simulink model "transmission_fault_detection"  (R2022b)
settings: Solver=VariableStepAuto  StartTime=0.0  StopTime=Tend  RelTol=1e-3  AbsTol=1e-3
PreLoadFcn:
  | Tend= 40;
  | numClutches= 6;
  | g1= 1.6; % Planetary ring/sun gear ratio
  | g2= 2.35; % Ravigneaux ring/large sun gear ratio
  | g3= 2.65; % Ravigneaux ring/small sun gear ratio
  | 
  | clutch_DR_table= [...
  | 0	0	0	0	0	0	0
  | 0	0	0	0	0	1	0
  | 0	0	0	0	1	0	0
  | 0	0	0	0	1	1	0
  | 0	0	0	1	0	0	0
  | 0	0	0	1	0	1	0
  | 0	0	0	1	1	0	0
  | 0	0	0	1	1	1	0
  | 0	0	1	0	0	0	0.002917
  | 0	0	1	0	0	1	0.004564
  | 0	0	1	0	1	0	0.009493
  | 0	0	1	0	1	1	0.412308
  | 0	0	1	1	0	0	0.011091
  | 0	0	1	1	0	1	0.232221
  | 0	0	1	1	1	0	0
  | 0	1	0	0	0	0	0.012267
  | 0	1	0	0	0	1	0.009497
  | 0	1	0	0	1	0	1.425532
  | 0	1	0	0	1	1	1.425532
  | 0	1	1	0	0	0	0.095756
  | 0	1	1	0	0	1	0.854862
  | 0	1	1	0	1	0	1.425532
  | 1	0	0	0	0	0	0.0001000
  | 1	0	0	0	0	1	0.0001100
  | 1	0	0	0	1	0	0
  | 1	0	0	1	0	0	-0.009327
  | 1	0	0	1	0	1	-0.261866
  | 1	0	0	1	1	0	0
  | 1	0	1	0	0	0	0.005888
  | 1	0	1	0	0	1	0.615385
  | 1	0	1	0	1	0	0
  | 1	0	1	1	0	0	0
  | 1	1	0	0	0	0	0.116338
  | 1	1	0	0	0	1	1.163666
  | 1	1	0	0	1	0	1.425532
  | 1	1	1	0	0	0	1];
libraries: fl_lib x19, nesl_utility x10, sdl_lib x8, simulink x4, matrix_library x1
CloseFcn:
  | clear clutch_DR_table numClutches g1 g2 g3 Tend simlog_sdl_transmission_fault_detection
  | clear logsout yout tout
  | try,close(h1_sdl_transmission_fault_detection),end
  | clear h1_sdl_transmission_fault_detection
Description:
  | Transmission Fault Detection
settings Model: PauseTimes=1  Creator=The MathWorks, Inc.  LastModifiedBy=lwh
settings SolverCC: AutoScaleAbsTol=off  MaxConsecutiveZCs=100  AlgebraicLoopSolver=TrustRegion  MaxZcPerStep=1
settings DataIOCC: ReturnWorkspaceOutputs=off
settings DebuggingCC: UnconnectedInputMsg=warning  UnconnectedOutputMsg=warning  UnconnectedLineMsg=warning  SymbolicDimsDataTypeCodeGenerationDiagnostic=none  SFMachineParentedDataDiag=warning
settings ModelReferenceCC: EnableRefExpFcnMdlSchedulingChecks=on
settings SFSimCC: CustomCodeUndefinedFunction=UseInterfaceOnly
settings RTWCC: DLArmComputeVersion=19.05
settings SimscapeCC: SimscapeLogType=all  SimscapeLogSimulationStatistics=on  SimscapeLogName=simlog_transmission_fault_detection  SimscapeLogDataHistory=10000

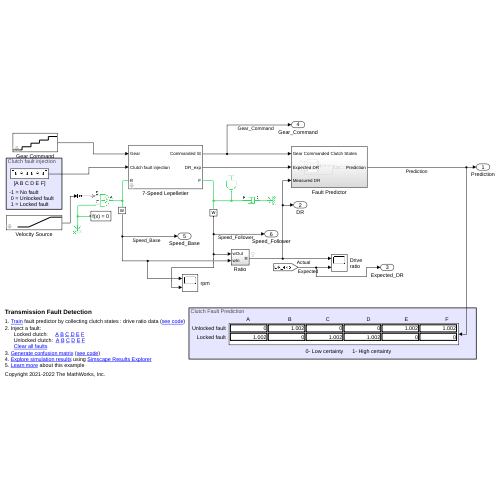
[thumbnail: Simulink's stored preview of the top-level diagram]
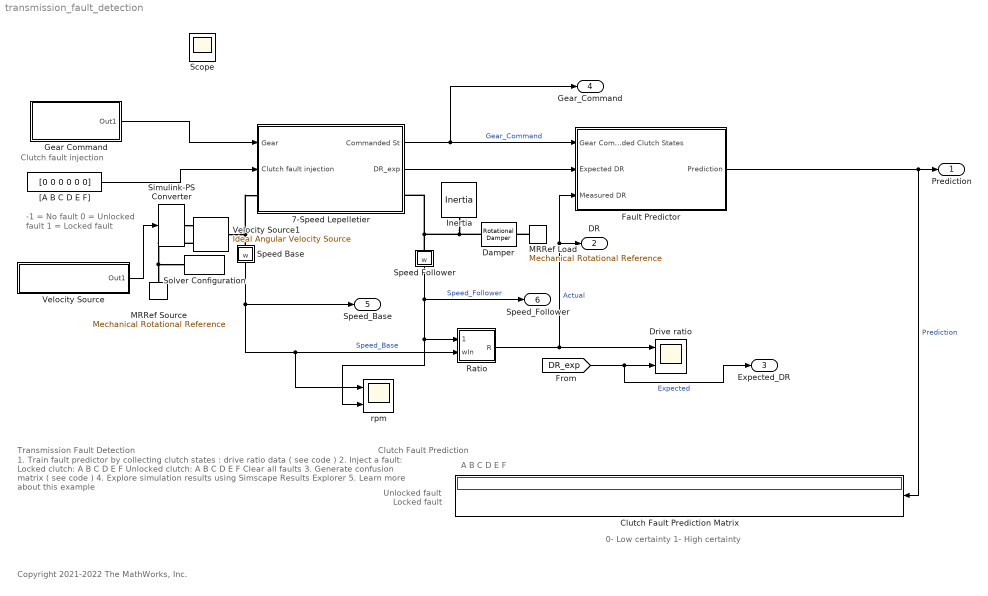
== system transmission_fault_detection ==
  note: Clutch fault injection
  note: -1 = No fault
      |  0 = Unlocked fault
      |  1 = Locked fault
  note: Locked fault
  note: 0- Low certainty 1- High certainty
  note: 1. Train fault predictor by collecting clutch states : drive ratio data ( see code )
      | 2. Inject a fault:
      | Locked clutch: A B C D E F
      | Unlocked clutch: A B C D E F
      | Clear all faults
      | 3. Generate confusion matrix ( see code )
      | 4. Explore simulation results using Simscape Results Explorer
      | 5. Learn more about this example
  note: A B C D E F
  note: Unlocked fault
  note: Transmission Fault Detection
  note: Clutch Fault Prediction
  note: Copyright 2021-2022 The MathWorks, Inc.
  7-Speed Lepelletier : Subsystem  mask(7-Speed Lepelletier){InitGear=Neutral, ShowInLibBrowser=0, ClutchSchedule={[0 1 0 0 1 1];[1 1 0 0 0 1];[1 1 1 0 0 0];[0 1 1 0 0 1];[1 0 1 0 0 1];[0 0 1 0 1 1];[0 0 1 1 0 1];[1 0 0 1 0 1];[0 0 0 1 0 1]}}
      mask prompts: InitGear "Initial gear"
      mask help: physmod:sdl:library:transmissions:SevenSpeedLepelletier
      mask init:
      | set_param([gcb,'/Clutch A'],'initial_state_locked',num2str(ClutchSchedule{InitGear}(1)));
      | set_param([gcb,'/Clutch B'],'initial_state_locked',num2str(ClutchSchedule{InitGear}(2)));
      | set_param([gcb,'/Clutch C'],'initial_state_locked',num2str(ClutchSchedule{InitGear}(3)));
      | set_param([gcb,'/Clutch D'],'initial_state_locked',num2str(ClutchSchedule{InitGear}(4)));
      | set_param([gcb,'/Clutch E'],'initial_state_locked',num2str(ClutchSchedule{InitGear}(5)));
      | set_param([gcb,'/Clutch F'],'initial_state_locked',num2str(ClutchSchedule{InitGear}(6)));
      mask Help: web([docroot '/sdl/ref/7speedlepelletier.html'])
      mask TypeOptions InitGear: 7 | 6 | 5 | 4 | 3 | 2 | 1 | physmod:sdl:library:transmissions:Reverse | physmod:sdl:library:transmissions:Neutral
  Clutch Fault Prediction Matrix : Display
  Damper : fl_lib/Mechanical/Rotational Elements/Rotational Damper  D=5 N*m/(rad/s)  w_specify=off  w_priority=High  w=0 rad/s  w_nominal_specify=off  w_nominal_unit=rad/s  w_nominal_value=1  t_specify=off  t_priority=High  t=0 N*m  t_nominal_specify=off  t_nominal_unit=N*m  t_nominal_value=1
  Drive ratio : Scope  NumInputPorts=2
  Fault Predictor : Subsystem
  Gear Command : Subsystem  mask{Repeating_Sequence=[7 7 7 7 7 7 7 7 7 7 7], Sample_time=4}
      mask prompts: Repeating_Sequence "Output"; Sample_time "Sample time"
      mask Display:
      | plot(0, -10)
      | plot(100, 100)
      | plot([0 20 20 40 40 60 60 80 80 100], [0 0 20 20 40 40 60 60 80 80]);
  Inertia : fl_lib/Mechanical/Rotational Elements/Inertia  inertia=.01 kg*m^2  num_ports=foundation.enum.numPorts2.one  w_specify=off  w_priority=High  w=0 rad/s  w_nominal_specify=off  w_nominal_unit=rad/s  w_nominal_value=1  t_specify=off  t_priority=High  t=0 N*m  t_nominal_specify=off  t_nominal_unit=N*m  t_nominal_value=1
  MRRef Load : fl_lib/Mechanical/Rotational Elements/Mechanical Rotational Reference
  MRRef Source : fl_lib/Mechanical/Rotational Elements/Mechanical Rotational Reference
  Ratio : Subsystem
  Simulink-PS Converter : nesl_utility/Simulink-PS Converter  PhysicalDomain=network_engine_domain  SubClassName=ps_input  LeftPortType=input  RightPortType=output  PseudoPeriodic=off  Frequencies=[]  NoiseDistribution=none  NoiseParameters=[]  Unit=rpm  AffineConversion=off  FilteringAndDerivatives=filter  SimscapeFilterOrder=1  InputFilterTimeConstant=0.001  UdotUserProvided=1
  Solver Configuration : nesl_utility/Solver Configuration  PhysicalDomain=network_engine_domain  SubClassName=solver  LeftPortType=input  RightPortType=generic  Tones=[]  Harmonics=[]  SimulateNoise=off  Profile=off  UseLocalSampling=off  EnableSwitchedLinearOptims=on  FrequencyDomain=off  UseCCode=off  RelTol=0.001  AbsTol=1e-06  MinStep=1e-09  ToWorkspace=off  RevertToSquareIcSolve=off  NumHomotopyIterations=100  PhasorMode=off  PhasorModeNumHarmonics=1  ConsistencySolver=NEWTON_XTOL_AFTER_FTOL  IndexReductionMethod=DerivativeReplacement  DoDC=on  ResidualTolerance=1e-9  ConsistencyTolSource=GLOBAL  ConsistencyAbsTol=0.001  ConsistencyRelTol=0.001  ConsistencyTolFactor=0.001  UseLocalSolver=off  LocalSolverChoice=NE_PARTITIONING_ADVANCER  ResolveIndetEquations=on  FunctionEvalNumThread=1  LocalSolverSampleTime=0.001  DoFixedCost=off  MaxNonlinIter=3  MaxModeIter=2  ComputeImpulses=off  ImpulseIterations=2  LinearAlgebra=auto  LinearAlgebraNumThread=0  EquationFormulation=NE_TIME_EF  DelaysMemoryBudget=1024  AutomaticFiltering=on  FilteringTimeConstant=0.001  PartitionStorageMethod=EXHAUSTIVE  PartitionMemoryBudget=1024  PartitionMethod=ROBUST
  Speed Base : Subsystem
      mask Display: disp('w')
  Speed Follower : Subsystem
      mask Display: disp('w')
  Velocity Source1 : fl_lib/Mechanical/Mechanical Sources/Ideal Angular Velocity Source
  Velocity Source : Subsystem  VariantControl=Ramp  mask{slope=100, start=0.1, initial_speed=450, final_speed=450}
      mask prompts: slope "Slope (rpm/s)"; start "Start time (sec)"; initial_speed "Initial speed (rpm)"; final_speed "Final speed (rpm)"
      mask Display:
      | plot(0, 0)
      | plot(100, 100)
      | plot([20 40 80 100], [20 20 90 90]);
  "[A B C D E F]" : Constant  Value=[0 0 0 0 0 0]  VectorParams1D=off
  rpm : Scope  NumInputPorts=2
  Prediction : Outport
  DR : Outport  Port=2
  Expected_DR : Outport  Port=3
  Gear_Command : Outport  Port=4
  Speed_Base : Outport  Port=5
  Speed_Follower : Outport  Port=6
  Scope : Scope
  wires:
  Fault Predictor/1(Prediction) -> Prediction/1, Clutch Fault Prediction Matrix/1  "Prediction"
  7-Speed Lepelletier/2(DR_exp) -> Fault Predictor/2(Expected DR)
  7-Speed Lepelletier/1(Commanded St) -> Gear_Command/1, Fault Predictor/1(Gear Commanded Clutch States)  "Gear_Command"
  Speed Base/1(w) -> Speed_Base/1, rpm/1, Ratio/2(wIn)  "Speed_Base"
  Speed Follower/1(w) -> Speed_Follower/1, rpm/2, Ratio/1(wOut)  "Speed_Follower"
  "[A B C D E F]"/1 -> 7-Speed Lepelletier/2(Clutch fault injection)
  Ratio/1(R) -> DR/1, Fault Predictor/3(Measured DR), Drive ratio/1  "Actual"
  [DR_exp] -> Expected_DR/1, Drive ratio/2  "Expected"
  Velocity Source/1(Out1) -> Simulink-PS Converter/1
  Gear Command/1(Out1) -> 7-Speed Lepelletier/1(Gear)
  connections:
  Velocity Source1/RConn2 -- MRRef Source/LConn1 -- Solver Configuration/RConn1
  Damper/LConn1 -- Inertia/LConn1 -- Speed Follower/LConn1 -- 7-Speed Lepelletier/RConn1
  Speed Base/LConn1 -- 7-Speed Lepelletier/LConn1 -- Velocity Source1/LConn1
  Simulink-PS Converter/RConn1 -- Velocity Source1/RConn1
  MRRef Load/LConn1 -- Damper/RConn1

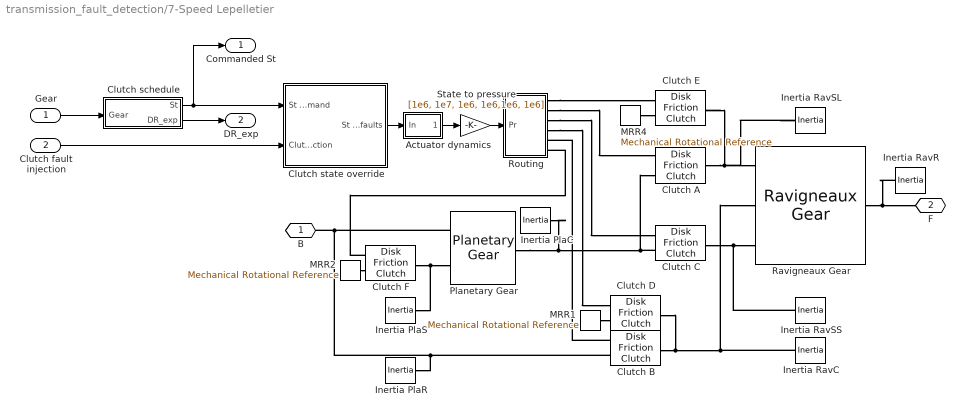
== system transmission_fault_detection/7-Speed Lepelletier ==
  Gear : Inport
  Clutch fault injection : Inport  Port=2
  Actuator dynamics : Subsystem  mask(First-order lag supporting vector signals){b=[1 1 1 1 1 1]*0.05, x_initial=ClutchSchedule{InitGear}}
      mask prompts: b "Filter time constant"; x_initial "Initial output"
      mask help: Models a lag of the form 1/(b*s+1) where s is the Laplace operator.
  Clutch schedule : Subsystem
  Clutch A : sdl_lib/Clutches/Disk Friction Clutch  geometry_model=2  r_eff=130 mm  d_o=150 mm  d_i=100 mm  nS=4  piston_area=0.001 m^2  unidirectional=0  friction_model=1  mu_w_vector=[ 0 0.1 0.2 0.3 0.4 0.5 1 2 5 10 100 1000 ] rad/s  temperature_TLU=[280.0, 300.0, 320.0] K  mu_static=0.65  mu_static_vector=[0.4, 0.38, 0.36]  mu_coulomb=0.6  mu_coulomb_vector=[ 0.29 0.28 0.26 0.22 0.21 0.2 0.2 0.19 0.19 0.19 0.19 0.19 ]  mu_coulomb_temp_vector=[0.3, 0.28, 0.25]  mu_coulomb_matrix=[0.34, 0.32, 0.3; 0.3, 0.28, 0.25; 0.25, 0.2, 0.15]  mu_interp_method=1  mu_extrap_method=1  d_f=1  w_tol=0.001 rad/s  pressure_min=100 Pa  mu_visc=0 N*m/(rad/s)  initial_state_locked=0  enable_faults=simscape.enum.onoff.off  fault_type=sdl.enum.clutchFault.lock  external_fault=simscape.enum.onoff.on  temporal_fault=simscape.enum.onoff.off  fault_time=5 s  report_fault=simscape.enum.assert.action.none  thermal_mass=25 kJ/K  T_init=300 K
      settings: InternalSimscapePortConfiguration="{\"Bottom\":[],\"Left\":[{\"id\":\"P\",\"label\":\"P\",\"type\":\"input\"},{\"id\":\"B\",\"label\":\"B\",\"type\":\"foundation.mechanical.rotational.rotational\"}],\"Right\":[{\"id\":\"F\",\"label\":\"F\",\"type\":\"foundation.mechanical.rotational.rotational\"}],\"Top\":[]}"
  Clutch B : sdl_lib/Clutches/Disk Friction Clutch  geometry_model=2  r_eff=130 mm  d_o=150 mm  d_i=100 mm  nS=4  piston_area=0.001 m^2  unidirectional=0  friction_model=1  mu_w_vector=[ 0 0.1 0.2 0.3 0.4 0.5 1 2 5 10 100 1000 ] rad/s  temperature_TLU=[280.0, 300.0, 320.0] K  mu_static=0.65  mu_static_vector=[0.4, 0.38, 0.36]  mu_coulomb=0.6  mu_coulomb_vector=[ 0.29 0.28 0.26 0.22 0.21 0.2 0.2 0.19 0.19 0.19 0.19 0.19 ]  mu_coulomb_temp_vector=[0.3, 0.28, 0.25]  mu_coulomb_matrix=[0.34, 0.32, 0.3; 0.3, 0.28, 0.25; 0.25, 0.2, 0.15]  mu_interp_method=1  mu_extrap_method=1  d_f=1  w_tol=0.001 rad/s  pressure_min=100 Pa  mu_visc=0 N*m/(rad/s)  initial_state_locked=0  enable_faults=simscape.enum.onoff.off  fault_type=sdl.enum.clutchFault.lock  external_fault=simscape.enum.onoff.off  temporal_fault=simscape.enum.onoff.off  fault_time=5 s  report_fault=simscape.enum.assert.action.none  thermal_mass=25 kJ/K  T_init=300 K
      settings: InternalSimscapePortConfiguration="{\"Bottom\":[],\"Left\":[{\"id\":\"P\",\"label\":\"P\",\"type\":\"input\"},{\"id\":\"B\",\"label\":\"B\",\"type\":\"foundation.mechanical.rotational.rotational\"}],\"Right\":[{\"id\":\"F\",\"label\":\"F\",\"type\":\"foundation.mechanical.rotational.rotational\"}],\"Top\":[]}"
  Clutch C : sdl_lib/Clutches/Disk Friction Clutch  geometry_model=2  r_eff=130 mm  d_o=150 mm  d_i=100 mm  nS=4  piston_area=0.001 m^2  unidirectional=0  friction_model=1  mu_w_vector=[ 0 0.1 0.2 0.3 0.4 0.5 1 2 5 10 100 1000 ] rad/s  temperature_TLU=[280.0, 300.0, 320.0] K  mu_static=0.65  mu_static_vector=[0.4, 0.38, 0.36]  mu_coulomb=0.6  mu_coulomb_vector=[ 0.29 0.28 0.26 0.22 0.21 0.2 0.2 0.19 0.19 0.19 0.19 0.19 ]  mu_coulomb_temp_vector=[0.3, 0.28, 0.25]  mu_coulomb_matrix=[0.34, 0.32, 0.3; 0.3, 0.28, 0.25; 0.25, 0.2, 0.15]  mu_interp_method=1  mu_extrap_method=1  d_f=1  w_tol=0.001 rad/s  pressure_min=100 Pa  mu_visc=0 N*m/(rad/s)  initial_state_locked=0  enable_faults=simscape.enum.onoff.off  fault_type=sdl.enum.clutchFault.lock  external_fault=simscape.enum.onoff.off  temporal_fault=simscape.enum.onoff.off  fault_time=5 s  report_fault=simscape.enum.assert.action.none  thermal_mass=25 kJ/K  T_init=300 K
      settings: InternalSimscapePortConfiguration="{\"Bottom\":[],\"Left\":[{\"id\":\"P\",\"label\":\"P\",\"type\":\"input\"},{\"id\":\"B\",\"label\":\"B\",\"type\":\"foundation.mechanical.rotational.rotational\"}],\"Right\":[{\"id\":\"F\",\"label\":\"F\",\"type\":\"foundation.mechanical.rotational.rotational\"}],\"Top\":[]}"
  Clutch D : sdl_lib/Clutches/Disk Friction Clutch  geometry_model=2  r_eff=130 mm  d_o=150 mm  d_i=100 mm  nS=4  piston_area=0.001 m^2  unidirectional=0  friction_model=1  mu_w_vector=[ 0 0.1 0.2 0.3 0.4 0.5 1 2 5 10 100 1000 ] rad/s  temperature_TLU=[280.0, 300.0, 320.0] K  mu_static=0.65  mu_static_vector=[0.4, 0.38, 0.36]  mu_coulomb=0.6  mu_coulomb_vector=[ 0.29 0.28 0.26 0.22 0.21 0.2 0.2 0.19 0.19 0.19 0.19 0.19 ]  mu_coulomb_temp_vector=[0.3, 0.28, 0.25]  mu_coulomb_matrix=[0.34, 0.32, 0.3; 0.3, 0.28, 0.25; 0.25, 0.2, 0.15]  mu_interp_method=1  mu_extrap_method=1  d_f=1  w_tol=0.001 rad/s  pressure_min=100 Pa  mu_visc=0 N*m/(rad/s)  initial_state_locked=1  enable_faults=simscape.enum.onoff.off  fault_type=sdl.enum.clutchFault.lock  external_fault=simscape.enum.onoff.off  temporal_fault=simscape.enum.onoff.off  fault_time=5 s  report_fault=simscape.enum.assert.action.none  thermal_mass=25 kJ/K  T_init=300 K
      settings: InternalSimscapePortConfiguration="{\"Bottom\":[],\"Left\":[{\"id\":\"P\",\"label\":\"P\",\"type\":\"input\"},{\"id\":\"B\",\"label\":\"B\",\"type\":\"foundation.mechanical.rotational.rotational\"}],\"Right\":[{\"id\":\"F\",\"label\":\"F\",\"type\":\"foundation.mechanical.rotational.rotational\"}],\"Top\":[]}"
  Clutch E : sdl_lib/Clutches/Disk Friction Clutch  geometry_model=2  r_eff=130 mm  d_o=150 mm  d_i=100 mm  nS=4  piston_area=0.001 m^2  unidirectional=0  friction_model=1  mu_w_vector=[ 0 0.1 0.2 0.3 0.4 0.5 1 2 5 10 100 1000 ] rad/s  temperature_TLU=[280.0, 300.0, 320.0] K  mu_static=0.65  mu_static_vector=[0.4, 0.38, 0.36]  mu_coulomb=0.6  mu_coulomb_vector=[ 0.29 0.28 0.26 0.22 0.21 0.2 0.2 0.19 0.19 0.19 0.19 0.19 ]  mu_coulomb_temp_vector=[0.3, 0.28, 0.25]  mu_coulomb_matrix=[0.34, 0.32, 0.3; 0.3, 0.28, 0.25; 0.25, 0.2, 0.15]  mu_interp_method=1  mu_extrap_method=1  d_f=1  w_tol=0.001 rad/s  pressure_min=100 Pa  mu_visc=0 N*m/(rad/s)  initial_state_locked=0  enable_faults=simscape.enum.onoff.off  fault_type=sdl.enum.clutchFault.lock  external_fault=simscape.enum.onoff.off  temporal_fault=simscape.enum.onoff.off  fault_time=5 s  report_fault=simscape.enum.assert.action.none  thermal_mass=25 kJ/K  T_init=300 K
      settings: InternalSimscapePortConfiguration="{\"Bottom\":[],\"Left\":[{\"id\":\"P\",\"label\":\"P\",\"type\":\"input\"},{\"id\":\"B\",\"label\":\"B\",\"type\":\"foundation.mechanical.rotational.rotational\"}],\"Right\":[{\"id\":\"F\",\"label\":\"F\",\"type\":\"foundation.mechanical.rotational.rotational\"}],\"Top\":[]}"
  Clutch F : sdl_lib/Clutches/Disk Friction Clutch  geometry_model=2  r_eff=130 mm  d_o=150 mm  d_i=100 mm  nS=4  piston_area=0.001 m^2  unidirectional=0  friction_model=1  mu_w_vector=[ 0 0.1 0.2 0.3 0.4 0.5 1 2 5 10 100 1000 ] rad/s  temperature_TLU=[280.0, 300.0, 320.0] K  mu_static=0.65  mu_static_vector=[0.4, 0.38, 0.36]  mu_coulomb=0.6  mu_coulomb_vector=[ 0.29 0.28 0.26 0.22 0.21 0.2 0.2 0.19 0.19 0.19 0.19 0.19 ]  mu_coulomb_temp_vector=[0.3, 0.28, 0.25]  mu_coulomb_matrix=[0.34, 0.32, 0.3; 0.3, 0.28, 0.25; 0.25, 0.2, 0.15]  mu_interp_method=1  mu_extrap_method=1  d_f=1  w_tol=0.001 rad/s  pressure_min=100 Pa  mu_visc=0 N*m/(rad/s)  initial_state_locked=1  enable_faults=simscape.enum.onoff.off  fault_type=sdl.enum.clutchFault.lock  external_fault=simscape.enum.onoff.off  temporal_fault=simscape.enum.onoff.off  fault_time=5 s  report_fault=simscape.enum.assert.action.none  thermal_mass=25 kJ/K  T_init=300 K
      settings: InternalSimscapePortConfiguration="{\"Bottom\":[],\"Left\":[{\"id\":\"P\",\"label\":\"P\",\"type\":\"input\"},{\"id\":\"B\",\"label\":\"B\",\"type\":\"foundation.mechanical.rotational.rotational\"}],\"Right\":[{\"id\":\"F\",\"label\":\"F\",\"type\":\"foundation.mechanical.rotational.rotational\"}],\"Top\":[]}"
  Clutch state override : Subsystem
  Inertia PlaC : fl_lib/Mechanical/Rotational Elements/Inertia  inertia=0.03 kg*m^2  num_ports=foundation.enum.numPorts2.one  w_specify=off  w_priority=High  w=0 rad/s  w_nominal_specify=off  w_nominal_unit=rad/s  w_nominal_value=1  t_specify=off  t_priority=High  t=0 N*m  t_nominal_specify=off  t_nominal_unit=N*m  t_nominal_value=1
  "Inertia PlaR " : fl_lib/Mechanical/Rotational Elements/Inertia  inertia=0.025 kg*m^2  num_ports=foundation.enum.numPorts2.one  w_specify=off  w_priority=High  w=0 rad/s  w_nominal_specify=off  w_nominal_unit=rad/s  w_nominal_value=1  t_specify=off  t_priority=High  t=0 N*m  t_nominal_specify=off  t_nominal_unit=N*m  t_nominal_value=1
  Inertia PlaS : fl_lib/Mechanical/Rotational Elements/Inertia  inertia=0.04 kg*m^2  num_ports=foundation.enum.numPorts2.one  w_specify=off  w_priority=High  w=0 rad/s  w_nominal_specify=off  w_nominal_unit=rad/s  w_nominal_value=1  t_specify=off  t_priority=High  t=0 N*m  t_nominal_specify=off  t_nominal_unit=N*m  t_nominal_value=1
  Inertia RavC : fl_lib/Mechanical/Rotational Elements/Inertia  inertia=0.03 kg*m^2  num_ports=foundation.enum.numPorts2.one  w_specify=off  w_priority=High  w=0 rad/s  w_nominal_specify=off  w_nominal_unit=rad/s  w_nominal_value=1  t_specify=off  t_priority=High  t=0 N*m  t_nominal_specify=off  t_nominal_unit=N*m  t_nominal_value=1
  Inertia RavR : fl_lib/Mechanical/Rotational Elements/Inertia  inertia=0.03 kg*m^2  num_ports=foundation.enum.numPorts2.one  w_specify=off  w_priority=High  w=0 rad/s  w_nominal_specify=off  w_nominal_unit=rad/s  w_nominal_value=1  t_specify=off  t_priority=High  t=0 N*m  t_nominal_specify=off  t_nominal_unit=N*m  t_nominal_value=1
  Inertia RavSL : fl_lib/Mechanical/Rotational Elements/Inertia  inertia=0.05 kg*m^2  num_ports=foundation.enum.numPorts2.one  w_specify=off  w_priority=High  w=0 rad/s  w_nominal_specify=off  w_nominal_unit=rad/s  w_nominal_value=1  t_specify=off  t_priority=High  t=0 N*m  t_nominal_specify=off  t_nominal_unit=N*m  t_nominal_value=1
  Inertia RavSS : fl_lib/Mechanical/Rotational Elements/Inertia  inertia=0.02 kg*m^2  num_ports=foundation.enum.numPorts2.one  w_specify=off  w_priority=High  w=0 rad/s  w_nominal_specify=off  w_nominal_unit=rad/s  w_nominal_value=1  t_specify=off  t_priority=High  t=0 N*m  t_nominal_specify=off  t_nominal_unit=N*m  t_nominal_value=1
  MRR1 : fl_lib/Mechanical/Rotational Elements/Mechanical Rotational Reference
  MRR2 : fl_lib/Mechanical/Rotational Elements/Mechanical Rotational Reference
  MRR4 : fl_lib/Mechanical/Rotational Elements/Mechanical Rotational Reference
  Planetary Gear : sdl_lib/Gears/Planetary Gear  rs_ratio=g1  friction_model=1  efficiency=[ 0.96 0.98 ]  temperature_TLU=[ 280 300 320 ] K  efficiency_sp_TLU=[ 0.95 0.9 0.85 ]  efficiency_rp_TLU=[ 0.95 0.9 0.85 ]  pwr_thr=[ 0.001 0.001 ] W  mu_visc=[ 0 0 ] N*m/(rad/s)  model_inertia=0  planet_inertia=0.001 kg*m^2  thermal_mass=50 J/K  T_init=300 K
  Ravigneaux Gear : sdl_lib/Gears/Ravigneaux Gear  rsl_ratio=g2  rss_ratio=g3  friction_model=1  efficiency=[ 0.98 0.98 0.98 0.99 ]  temperature_TLU=[ 280 300 320 ] K  efficiency_lsp_TLU=[ 0.95 0.9 0.85 ]  efficiency_ssp_TLU=[ 0.95 0.9 0.85 ]  efficiency_rp_TLU=[ 0.95 0.9 0.85 ]  efficiency_pp_TLU=[ 0.95 0.9 0.85 ]  pwr_thr=[ 0.001 0.001 0.001 0.001 ] W  mu_visc=[ 0 0 0 0 ] N*m/(rad/s)  model_inertia=0  inner_planet_inertia=0.001 kg*m^2  outer_planet_inertia=0.001 kg*m^2  thermal_mass=50 J/K  T_init=300 K
      settings: InternalSimscapePortConfiguration="{\"Bottom\":[],\"Left\":[{\"id\":\"SL\",\"label\":\"SL\",\"type\":\"foundation.mechanical.rotational.rotational\"},{\"id\":\"C\",\"label\":\"C\",\"type\":\"foundation.mechanical.rotational.rotational\"},{\"id\":\"SS\",\"label\":\"SS\",\"type\":\"foundation.mechanical.rotational.rotational\"}],\"Right\":[{\"id\":\"R\",\"label\":\"R\",\"type\":\"foundation.mechanical.rotational.rotational\"}],\"Top\":[]}"
  Routing : Subsystem
  State to pressure : Gain  Gain=[1e6, 1e7, 1e6, 1e6,1e6, 1e6]
  B : PMIOPort  Side=Left
  F : PMIOPort  Port=2  Side=Right
  Commanded St : Outport
  DR_exp : Outport  Port=2
  wires:
  Actuator dynamics/1(Out) -> State to pressure/1
  State to pressure/1 -> Routing/1(Pr)
  Gear/1 -> Clutch schedule/1(Gear)
  Clutch schedule/1(St) -> Clutch state override/1(St Command), Commanded St/1
  Clutch fault injection/1 -> Clutch state override/2(Clutch fault injection)
  Clutch state override/1(St with faults) -> Actuator dynamics/1(In)
  Clutch schedule/2(DR_exp) -> DR_exp/1
  connections:
  Clutch B/LConn2 -- Planetary Gear/RConn1 -- B/RConn1 -- "Inertia PlaR "/LConn1
  Inertia RavR/LConn1 -- Ravigneaux Gear/RConn1 -- F/RConn1
  Inertia PlaS/LConn1 -- Clutch F/RConn1 -- Planetary Gear/RConn2
  Inertia RavSS/LConn1 -- Clutch C/RConn1 -- Ravigneaux Gear/LConn3
  Clutch E/RConn1 -- Inertia RavSL/LConn1 -- Ravigneaux Gear/LConn1 -- Clutch A/RConn1
  Clutch D/RConn1 -- Clutch B/RConn1 -- Ravigneaux Gear/LConn2 -- Inertia RavC/LConn1
  Inertia PlaC/LConn1 -- Clutch C/LConn2 -- Clutch A/LConn2 -- Planetary Gear/LConn1
  Routing/RConn4 -- Clutch D/LConn1
  Clutch B/LConn1 -- Routing/RConn5
  Routing/RConn3 -- Clutch C/LConn1
  Routing/RConn2 -- Clutch A/LConn1
  MRR2/LConn1 -- Clutch F/LConn2
  Clutch F/LConn1 -- Routing/RConn6
  MRR1/LConn1 -- Clutch D/LConn2
  MRR4/LConn1 -- Clutch E/LConn2
  Routing/RConn1 -- Clutch E/LConn1

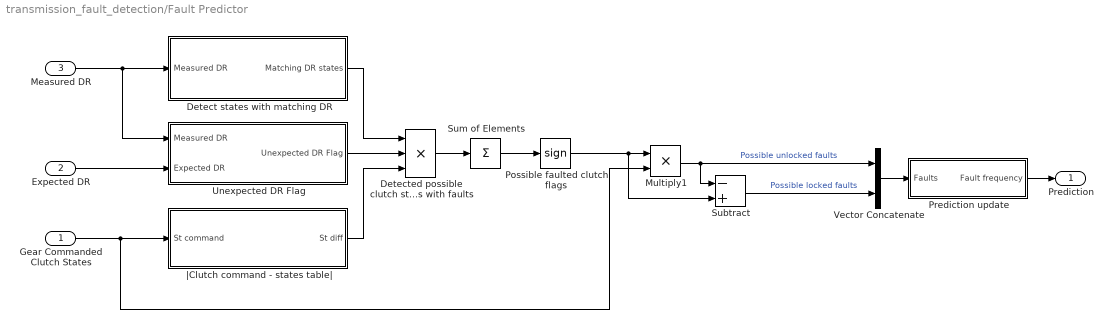
== system transmission_fault_detection/Fault Predictor ==
  Gear Commanded Clutch States : Inport  SampleTime=0.1
  Expected DR : Inport  Port=2  SampleTime=0.1
  Measured DR : Inport  Port=3  SampleTime=0.1
  Detect states with matching DR : Subsystem
  Detected possible clutch states with faults : Product  Inputs=***
  Multiply1 : Product  Inputs=**
  Possible faulted clutch flags : Signum
  Prediction update : Subsystem
  Subtract : Sum  Inputs=-+
  Sum of Elements : Sum  Inputs=+  CollapseMode=Specified dimension
  Unexpected DR Flag : Subsystem
  Vector Concatenate : Concatenate  Mode=Multidimensional array  ConcatenateDimension=2
  |Clutch command - states table| : Subsystem
  Prediction : Outport
  wires:
  Detected possible clutch states with faults/1 -> Sum of Elements/1
  Gear Commanded Clutch States/1 -> |Clutch command - states table|/1(St command), Multiply1/2
  Multiply1/1 -> Vector Concatenate/1, Subtract/1  "Possible unlocked faults"
  Measured DR/1 -> Unexpected DR Flag/1(Measured DR), Detect states with matching DR/1(Measured DR)
  Sum of Elements/1 -> Possible faulted clutch flags/1
  Vector Concatenate/1 -> Prediction update/1(Faults)
  |Clutch command - states table|/1(St diff) -> Detected possible clutch states with faults/3
  Detect states with matching DR/1(Matching DR states) -> Detected possible clutch states with faults/1
  Unexpected DR Flag/1(Unexpected DR Flag) -> Detected possible clutch states with faults/2
  Expected DR/1 -> Unexpected DR Flag/2(Expected DR)
  Subtract/1 -> Vector Concatenate/2  "Possible locked faults"
  Possible faulted clutch flags/1 -> Subtract/2, Multiply1/1
  Prediction update/1(Fault frequency) -> Prediction/1

== system transmission_fault_detection/Gear Command ==
  Gear Command : simulink/Sources/Repeating Sequence Stair  OutValues=Repeating_Sequence  tsamp=Sample_time  OutMin=[]  OutMax=[]  OutDataTypeStr=double  OutputDataTypeScalingMode=double  OutDataType=fixdt(0,8)  ConRadixGroup=Best Precision: Vector-wise  OutScaling=2^-12
  Out1 : Outport
  wires:
  Gear Command/1 -> Out1/1

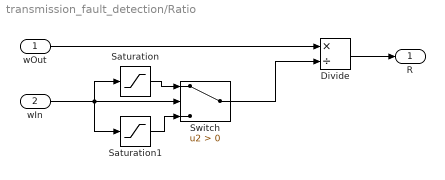
== system transmission_fault_detection/Ratio ==
  wOut : Inport
  wIn : Inport  Port=2
  Divide : Product  Inputs=*/
  Saturation : Saturate  UpperLimit=Inf  LowerLimit=1e-3  ZeroCross=off
  Saturation1 : Saturate  UpperLimit=-1e-3  LowerLimit=-Inf  ZeroCross=off
  Switch : Switch  Criteria=u2 > Threshold  ZeroCross=off  SaturateOnIntegerOverflow=off  InputSameDT=off
  R : Outport  VectorParamsAs1DForOutWhenUnconnected=off
  wires:
  wOut/1 -> Divide/1
  wIn/1 -> Saturation1/1, Saturation/1, Switch/2
  Divide/1 -> R/1
  Saturation/1 -> Switch/1
  Switch/1 -> Divide/2
  Saturation1/1 -> Switch/3

== system transmission_fault_detection/Speed Base ==
  MRRef : fl_lib/Mechanical/Rotational Elements/Mechanical Rotational Reference
  Motion Sensor : fl_lib/Mechanical/Mechanical Sensors/Ideal Rotational Motion Sensor  reference=foundation.enum.MeasurementReference.difference  acceleration_port=false  velocity_port=true  position_port=true  wrap_angle=simscape.enum.onoff.off  offset=0 rad
  PS-Simulink Converter1 : nesl_utility/PS-Simulink Converter  PhysicalDomain=network_engine_domain  SubClassName=ps_output  LeftPortType=input  RightPortType=output  PseudoPeriodic=off  Frequencies=[]  VectorFormat=1-D array  Unit=rad/s  AffineConversion=off
  R : PMIOPort  Side=Left
  w : Outport  VectorParamsAs1DForOutWhenUnconnected=off
  wires:
  PS-Simulink Converter1/1 -> w/1
  connections:
  MRRef/LConn1 -- Motion Sensor/RConn1
  Motion Sensor/RConn2 -- PS-Simulink Converter1/LConn1
  R/RConn1 -- Motion Sensor/LConn1

== system transmission_fault_detection/Speed Follower ==
  MRRef : fl_lib/Mechanical/Rotational Elements/Mechanical Rotational Reference
  Motion Sensor : fl_lib/Mechanical/Mechanical Sensors/Ideal Rotational Motion Sensor  reference=foundation.enum.MeasurementReference.difference  acceleration_port=false  velocity_port=true  position_port=true  wrap_angle=simscape.enum.onoff.off  offset=0 rad
  PS-Simulink Converter1 : nesl_utility/PS-Simulink Converter  PhysicalDomain=network_engine_domain  SubClassName=ps_output  LeftPortType=input  RightPortType=output  PseudoPeriodic=off  Frequencies=[]  VectorFormat=1-D array  Unit=rad/s  AffineConversion=off
  R : PMIOPort  Side=Left
  w : Outport  VectorParamsAs1DForOutWhenUnconnected=off
  wires:
  PS-Simulink Converter1/1 -> w/1  "Follower"
  connections:
  R/RConn1 -- Motion Sensor/LConn1
  Motion Sensor/RConn2 -- PS-Simulink Converter1/LConn1
  MRRef/LConn1 -- Motion Sensor/RConn1

== system transmission_fault_detection/Velocity Source ==
  Ramp : simulink/Sources/Ramp  slope=slope  start=start  InitialOutput=initial_speed
  Saturation : Saturate  UpperLimit=max(initial_speed, final_speed)  LowerLimit=min(initial_speed, final_speed)
  Out1 : Outport
  wires:
  Ramp/1 -> Saturation/1
  Saturation/1 -> Out1/1

== system transmission_fault_detection/7-Speed Lepelletier/Actuator dynamics ==
  In : Inport
  Gain : Gain  Gain=1./b
  Integrator : Integrator  InitialCondition=x_initial.*b
  Sum : Sum  Inputs=|+-  InputSameDT=on  SaturateOnIntegerOverflow=on  OutDataTypeStr=Inherit: Same as first input
  Out : Outport  VectorParamsAs1DForOutWhenUnconnected=off
  wires:
  Sum/1 -> Integrator/1
  In/1 -> Sum/1
  Integrator/1 -> Gain/1
  Gain/1 -> Sum/2, Out/1

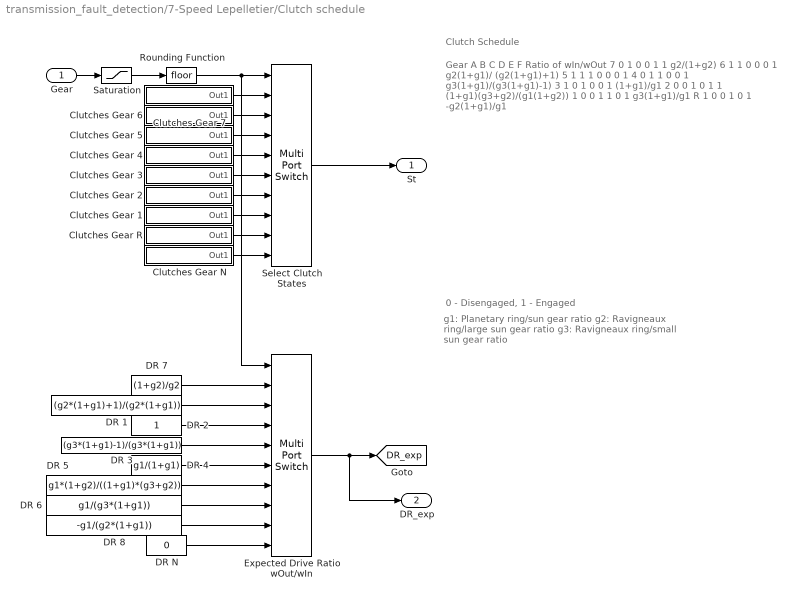
== system transmission_fault_detection/7-Speed Lepelletier/Clutch schedule ==
  note: Clutch Schedule
  note: Gear
      | A
      | B
      | C
      | D
      | E
      | F
      | Ratio of wIn/wOut
      |
      | 7
      | 0
      | 1
      | 0
      | 0
      | 1
      | 1
      | g2/(1+g2)
      |
      | 6
      | 1
      | 1
      | 0
      | 0
      | 0
      | 1
      | g2(1+g1)/ (g2(1+g1)+1)
      |
      | 5
      | 1
      | 1
      | 1
      | 0
      | 0
      | 0
      | 1
      |
      | 4
      | 0
      | 1
      | 1
      | 0
      | 0
      | 1
      | g3(1+g1)/(g3(1+g1)-1)
      |
      | 3
      | 1
      | 0
      | 1
      | 0
      | 0
      | 1
      | (1+g1)/g1
      |
      | 2
      | 0
      | 0
      | 1
      | 0
      | 1
      | 1
      | (1+g1)(g3+g2)/(g1(1+g2))
      |
      | 1
      | 0
      | 0
      | 1
      | 1
      | 0
      | 1
      | g3(1+g1)/g1
      |
      | R
      | 1
      | 0
      | 0
      | 1
      | 0
      | 1
      | -g2(1+g1)/g1
  note: 0 - Disengaged, 1 - Engaged
  note: g1: Planetary ring/sun gear ratio
      | g2: Ravigneaux ring/large sun gear ratio
      | g3: Ravigneaux ring/small sun gear ratio
  Gear : Inport
  Clutches Gear 1 : Subsystem  mask{Clutches=ClutchSchedule{7}}
      settings: OpenFcn=open_system(gcb,'force');
      mask Display: disp(Clutches)
  Clutches Gear 2 : Subsystem  mask{Clutches=ClutchSchedule{6}}
      settings: OpenFcn=open_system(gcb,'force');
      mask Display: disp(Clutches)
  Clutches Gear 3 : Subsystem  mask{Clutches=ClutchSchedule{5}}
      settings: OpenFcn=open_system(gcb,'force');
      mask Display: disp(Clutches)
  Clutches Gear 4 : Subsystem  mask{Clutches=ClutchSchedule{4}}
      settings: OpenFcn=open_system(gcb,'force');
      mask Display: disp(Clutches)
  Clutches Gear 5 : Subsystem  mask{Clutches=ClutchSchedule{3}}
      settings: OpenFcn=open_system(gcb,'force');
      mask Display: disp(Clutches)
  Clutches Gear 6 : Subsystem  mask{Clutches=ClutchSchedule{2}}
      settings: OpenFcn=open_system(gcb,'force');
      mask Display: disp(Clutches)
  Clutches Gear 7 : Subsystem  mask{Clutches=ClutchSchedule{1}}
      settings: OpenFcn=open_system(gcb,'force');
      mask Display: disp(Clutches)
  Clutches Gear N : Subsystem  mask{Clutches=ClutchSchedule{9}}
      settings: OpenFcn=open_system(gcb,'force');
      mask Display: disp(Clutches)
  Clutches Gear R : Subsystem  mask{Clutches=ClutchSchedule{8}}
      settings: OpenFcn=open_system(gcb,'force');
      mask Display: disp(Clutches)
  DR 1 : Constant  Value=(g2*(1+g1)+1)/(g2*(1+g1))
  DR 2 : Constant
  DR 3 : Constant  Value=(g3*(1+g1)-1)/(g3*(1+g1))
  DR 4 : Constant  Value=g1/(1+g1)
  DR 5 : Constant  Value=g1*(1+g2)/((1+g1)*(g3+g2))
  DR 6 : Constant  Value=g1/(g3*(1+g1))
  DR 7 : Constant  Value=(1+g2)/g2
  DR 8 : Constant  Value=-g1/(g2*(1+g1))
  DR N : Constant  Value=0
  "Expected Drive Ratio wOut/wIn " : MultiPortSwitch  DataPortOrder=Specify indices  DataPortIndices={7,6,5,4,3,2,1,-1,0}  DiagnosticForDefault=None  SaturateOnIntegerOverflow=off  InputSameDT=off
  Rounding Function : Rounding
  Saturation : Saturate  UpperLimit=7  LowerLimit=-1  ZeroCross=off
  Select Clutch States : MultiPortSwitch  DataPortOrder=Specify indices  DataPortIndices={7,6,5,4,3,2,1,-1,0}  DiagnosticForDefault=None  SaturateOnIntegerOverflow=off  InputSameDT=off
  St : Outport  VectorParamsAs1DForOutWhenUnconnected=off
  DR_exp : Outport  Port=2  VectorParamsAs1DForOutWhenUnconnected=off
  tag scope: DR_exp=global
  wires:
  Select Clutch States/1 -> St/1
  Gear/1 -> Saturation/1
  Clutches Gear N/1(Out1) -> Select Clutch States/10
  Saturation/1 -> Rounding Function/1
  Rounding Function/1 -> "Expected Drive Ratio wOut/wIn "/1, Select Clutch States/1
  Clutches Gear R/1(Out1) -> Select Clutch States/9
  Clutches Gear 1/1(Out1) -> Select Clutch States/8
  Clutches Gear 2/1(Out1) -> Select Clutch States/7
  Clutches Gear 3/1(Out1) -> Select Clutch States/6
  Clutches Gear 4/1(Out1) -> Select Clutch States/5
  Clutches Gear 5/1(Out1) -> Select Clutch States/4
  Clutches Gear 6/1(Out1) -> Select Clutch States/3
  Clutches Gear 7/1(Out1) -> Select Clutch States/2
  DR 6/1 -> "Expected Drive Ratio wOut/wIn "/8
  DR N/1 -> "Expected Drive Ratio wOut/wIn "/10
  DR 8/1 -> "Expected Drive Ratio wOut/wIn "/9
  DR 5/1 -> "Expected Drive Ratio wOut/wIn "/7
  "Expected Drive Ratio wOut/wIn "/1 -> DR_exp/1, [DR_exp]
  DR 7/1 -> "Expected Drive Ratio wOut/wIn "/2
  DR 1/1 -> "Expected Drive Ratio wOut/wIn "/3
  DR 2/1 -> "Expected Drive Ratio wOut/wIn "/4
  DR 3/1 -> "Expected Drive Ratio wOut/wIn "/5
  DR 4/1 -> "Expected Drive Ratio wOut/wIn "/6

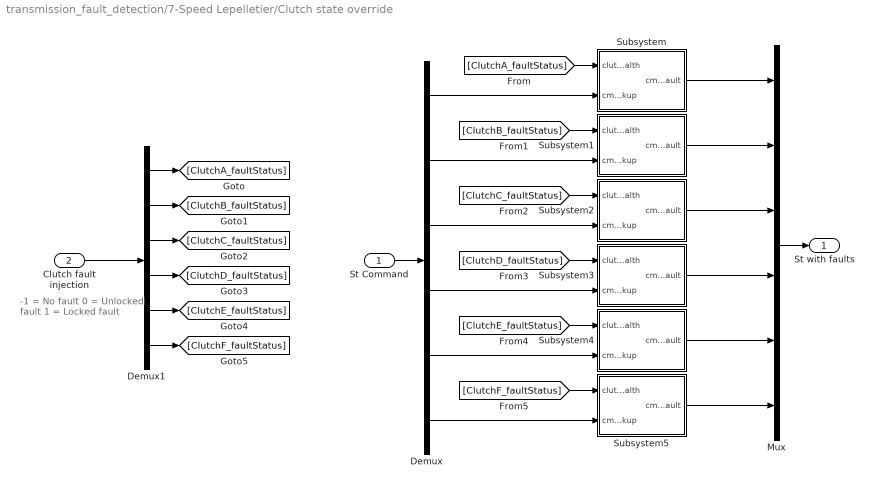
== system transmission_fault_detection/7-Speed Lepelletier/Clutch state override ==
  note: -1 = No fault
      |  0 = Unlocked fault
      | 1 = Locked fault
  St Command : Inport
  Clutch fault injection : Inport  Port=2
  Demux : Demux  Outputs=6
  Demux1 : Demux  Outputs=6
  Mux : Mux  Inputs=6
  Subsystem : Subsystem
  Subsystem1 : Subsystem
  Subsystem2 : Subsystem
  Subsystem3 : Subsystem
  Subsystem4 : Subsystem
  Subsystem5 : Subsystem
  St with faults : Outport  VectorParamsAs1DForOutWhenUnconnected=off
  wires:
  [ClutchF_faultStatus] -> Subsystem5/1(clutch_health)
  [ClutchE_faultStatus] -> Subsystem4/1(clutch_health)
  [ClutchD_faultStatus] -> Subsystem3/1(clutch_health)
  [ClutchC_faultStatus] -> Subsystem2/1(clutch_health)
  [ClutchB_faultStatus] -> Subsystem1/1(clutch_health)
  [ClutchA_faultStatus] -> Subsystem/1(clutch_health)
  Clutch fault injection/1 -> Demux1/1
  Demux1/6 -> [ClutchF_faultStatus]
  Demux1/5 -> [ClutchE_faultStatus]
  Demux1/4 -> [ClutchD_faultStatus]
  Demux1/3 -> [ClutchC_faultStatus]
  Demux1/2 -> [ClutchB_faultStatus]
  Demux1/1 -> [ClutchA_faultStatus]
  Subsystem5/1(cmd_wFault) -> Mux/6
  Subsystem4/1(cmd_wFault) -> Mux/5
  Subsystem/1(cmd_wFault) -> Mux/1
  Subsystem3/1(cmd_wFault) -> Mux/4
  Subsystem1/1(cmd_wFault) -> Mux/2
  Subsystem2/1(cmd_wFault) -> Mux/3
  Mux/1 -> St with faults/1
  Demux/6 -> Subsystem5/2(cmd_lookup)
  Demux/5 -> Subsystem4/2(cmd_lookup)
  Demux/4 -> Subsystem3/2(cmd_lookup)
  Demux/3 -> Subsystem2/2(cmd_lookup)
  Demux/2 -> Subsystem1/2(cmd_lookup)
  Demux/1 -> Subsystem/2(cmd_lookup)
  St Command/1 -> Demux/1

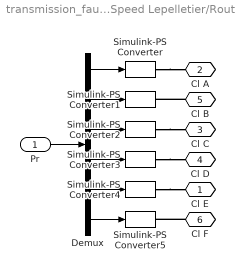
== system transmission_fault_detection/7-Speed Lepelletier/Routing ==
  Pr : Inport
  Demux : Demux  Outputs=6
  Simulink-PS Converter{,1..5} (6 alike) : nesl_utility/Simulink-PS Converter  PhysicalDomain=network_engine_domain  SubClassName=ps_input  LeftPortType=input  RightPortType=output  PseudoPeriodic=off  Frequencies=[]  NoiseDistribution=none  NoiseParameters=[]  Unit=1  AffineConversion=off  FilteringAndDerivatives=zero  SimscapeFilterOrder=1  InputFilterTimeConstant=0.001  UdotUserProvided=1
  Cl E : PMIOPort  Side=Right
  Cl A : PMIOPort  Port=2  Side=Right
  Cl C : PMIOPort  Port=3  Side=Right
  Cl D : PMIOPort  Port=4  Side=Right
  Cl B : PMIOPort  Port=5  Side=Right
  Cl F : PMIOPort  Port=6  Side=Right
  wires:
  Pr/1 -> Demux/1
  Demux/1 -> Simulink-PS Converter/1
  Demux/2 -> Simulink-PS Converter1/1
  Demux/6 -> Simulink-PS Converter5/1
  Demux/5 -> Simulink-PS Converter4/1
  Demux/4 -> Simulink-PS Converter3/1
  Demux/3 -> Simulink-PS Converter2/1
  connections:
  Simulink-PS Converter3/RConn1 -- Cl D/RConn1
  Simulink-PS Converter/RConn1 -- Cl A/RConn1
  Simulink-PS Converter4/RConn1 -- Cl E/RConn1
  Cl B/RConn1 -- Simulink-PS Converter1/RConn1
  Simulink-PS Converter2/RConn1 -- Cl C/RConn1
  Cl F/RConn1 -- Simulink-PS Converter5/RConn1

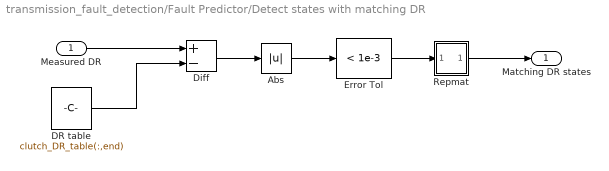
== system transmission_fault_detection/Fault Predictor/Detect states with matching DR ==
  Measured DR : Inport
  Abs : Abs  SaturateOnIntegerOverflow=off
  DR table : Constant  Value=clutch_DR_table(:,end)  SampleTime=0.1
  Diff : Sum  Inputs=+-
  Error Tol : simulink/Logic and Bit Operations/Compare To Constant  relop=<  const=1e-3  OutDataTypeStr=boolean
  Repmat : Subsystem
  Matching DR states : Outport
  wires:
  Diff/1 -> Abs/1
  Abs/1 -> Error Tol/1
  Error Tol/1 -> Repmat/1(In)
  DR table/1 -> Diff/2
  Repmat/1(Out) -> Matching DR states/1
  Measured DR/1 -> Diff/1

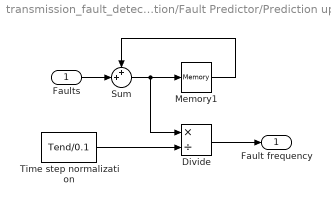
== system transmission_fault_detection/Fault Predictor/Prediction update ==
  Faults : Inport
  Divide : Product  Inputs=*/
  Memory1 : Memory  InheritSampleTime=on
  Sum : Sum  Inputs=++|
  Time step normalization : Constant  Value=Tend/0.1  SampleTime=0.1
  Fault frequency : Outport
  wires:
  Divide/1 -> Fault frequency/1
  Faults/1 -> Sum/2
  Memory1/1 -> Sum/1
  Sum/1 -> Divide/1, Memory1/1
  Time step normalization/1 -> Divide/2

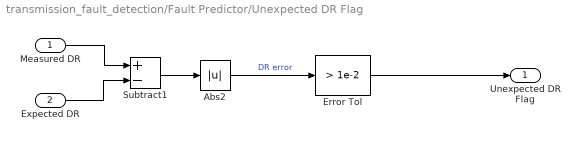
== system transmission_fault_detection/Fault Predictor/Unexpected DR Flag ==
  Measured DR : Inport
  Expected DR : Inport  Port=2
  Abs2 : Abs  SaturateOnIntegerOverflow=off
  Error Tol : simulink/Logic and Bit Operations/Compare To Constant  relop=>  const=1e-2  OutDataTypeStr=uint8
  Subtract1 : Sum  Inputs=+-
  Unexpected DR Flag : Outport
  wires:
  Abs2/1 -> Error Tol/1  "DR error"
  Subtract1/1 -> Abs2/1
  Expected DR/1 -> Subtract1/2
  Measured DR/1 -> Subtract1/1
  Error Tol/1 -> Unexpected DR Flag/1

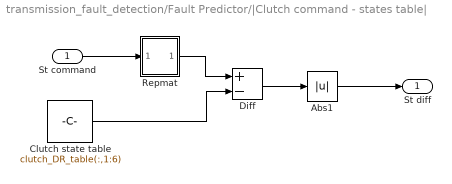
== system transmission_fault_detection/Fault Predictor/|Clutch command - states table| ==
  St command : Inport
  Abs1 : Abs  SaturateOnIntegerOverflow=off
  Clutch state table : Constant  Value=clutch_DR_table(:,1:6)  VectorParams1D=off  SampleTime=0.1
  Diff : Sum  Inputs=+-
  Repmat : Subsystem
  St diff : Outport
  wires:
  Abs1/1 -> St diff/1
  Repmat/1(Out1) -> Diff/1
  Clutch state table/1 -> Diff/2
  St command/1 -> Repmat/1(In1)
  Diff/1 -> Abs1/1

== system transmission_fault_detection/7-Speed Lepelletier/Clutch schedule/Clutches Gear 1 ==
  Clutches : Constant  Value=Clutches  SampleTime=0
  Out1 : Outport  VectorParamsAs1DForOutWhenUnconnected=off
  wires:
  Clutches/1 -> Out1/1

== system transmission_fault_detection/7-Speed Lepelletier/Clutch schedule/Clutches Gear 2 ==
  Clutches : Constant  Value=Clutches  SampleTime=0
  Out1 : Outport  VectorParamsAs1DForOutWhenUnconnected=off
  wires:
  Clutches/1 -> Out1/1

== system transmission_fault_detection/7-Speed Lepelletier/Clutch schedule/Clutches Gear 3 ==
  Clutches : Constant  Value=Clutches  SampleTime=0
  Out1 : Outport  VectorParamsAs1DForOutWhenUnconnected=off
  wires:
  Clutches/1 -> Out1/1

== system transmission_fault_detection/7-Speed Lepelletier/Clutch schedule/Clutches Gear 4 ==
  Clutches : Constant  Value=Clutches  SampleTime=0
  Out1 : Outport  VectorParamsAs1DForOutWhenUnconnected=off
  wires:
  Clutches/1 -> Out1/1

== system transmission_fault_detection/7-Speed Lepelletier/Clutch schedule/Clutches Gear 5 ==
  Clutches : Constant  Value=Clutches  SampleTime=0
  Out1 : Outport  VectorParamsAs1DForOutWhenUnconnected=off
  wires:
  Clutches/1 -> Out1/1

== system transmission_fault_detection/7-Speed Lepelletier/Clutch schedule/Clutches Gear 6 ==
  Clutches : Constant  Value=Clutches  SampleTime=0
  Out1 : Outport  VectorParamsAs1DForOutWhenUnconnected=off
  wires:
  Clutches/1 -> Out1/1

== system transmission_fault_detection/7-Speed Lepelletier/Clutch schedule/Clutches Gear 7 ==
  Clutches : Constant  Value=Clutches  SampleTime=0
  Out1 : Outport  VectorParamsAs1DForOutWhenUnconnected=off
  wires:
  Clutches/1 -> Out1/1

== system transmission_fault_detection/7-Speed Lepelletier/Clutch schedule/Clutches Gear N ==
  Clutches Gear N : Constant  Value=Clutches  SampleTime=0
  Out1 : Outport  VectorParamsAs1DForOutWhenUnconnected=off
  wires:
  Clutches Gear N/1 -> Out1/1

== system transmission_fault_detection/7-Speed Lepelletier/Clutch schedule/Clutches Gear R ==
  Clutches : Constant  Value=Clutches  SampleTime=0
  Out1 : Outport  VectorParamsAs1DForOutWhenUnconnected=off
  wires:
  Clutches/1 -> Out1/1

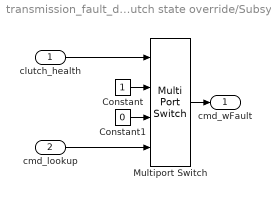
== system transmission_fault_detection/7-Speed Lepelletier/Clutch state override/Subsystem ==
  clutch_health : Inport
  cmd_lookup : Inport  Port=2
  Constant : Constant
  Constant1 : Constant  Value=0
  Multiport Switch : MultiPortSwitch  DataPortOrder=Specify indices  DataPortIndices={1,0,-1}  DiagnosticForDefault=None  SaturateOnIntegerOverflow=off  InputSameDT=off
  cmd_wFault : Outport
  wires:
  clutch_health/1 -> Multiport Switch/1
  Constant1/1 -> Multiport Switch/3
  Multiport Switch/1 -> cmd_wFault/1
  Constant/1 -> Multiport Switch/2
  cmd_lookup/1 -> Multiport Switch/4

== system transmission_fault_detection/7-Speed Lepelletier/Clutch state override/Subsystem1 ==
  clutch_health : Inport
  cmd_lookup : Inport  Port=2
  Constant : Constant
  Constant1 : Constant  Value=0
  Multiport Switch : MultiPortSwitch  DataPortOrder=Specify indices  DataPortIndices={1,0,-1}  DiagnosticForDefault=None  SaturateOnIntegerOverflow=off  InputSameDT=off
  cmd_wFault : Outport
  wires:
  cmd_lookup/1 -> Multiport Switch/4
  Constant/1 -> Multiport Switch/2
  Multiport Switch/1 -> cmd_wFault/1
  Constant1/1 -> Multiport Switch/3
  clutch_health/1 -> Multiport Switch/1

== system transmission_fault_detection/7-Speed Lepelletier/Clutch state override/Subsystem2 ==
  clutch_health : Inport
  cmd_lookup : Inport  Port=2
  Constant : Constant
  Constant1 : Constant  Value=0
  Multiport Switch : MultiPortSwitch  DataPortOrder=Specify indices  DataPortIndices={1,0,-1}  DiagnosticForDefault=None  SaturateOnIntegerOverflow=off  InputSameDT=off
  cmd_wFault : Outport
  wires:
  clutch_health/1 -> Multiport Switch/1
  Constant1/1 -> Multiport Switch/3
  Multiport Switch/1 -> cmd_wFault/1
  Constant/1 -> Multiport Switch/2
  cmd_lookup/1 -> Multiport Switch/4

== system transmission_fault_detection/7-Speed Lepelletier/Clutch state override/Subsystem3 ==
  clutch_health : Inport
  cmd_lookup : Inport  Port=2
  Constant : Constant
  Constant1 : Constant  Value=0
  Multiport Switch : MultiPortSwitch  DataPortOrder=Specify indices  DataPortIndices={1,0,-1}  DiagnosticForDefault=None  SaturateOnIntegerOverflow=off  InputSameDT=off
  cmd_wFault : Outport
  wires:
  cmd_lookup/1 -> Multiport Switch/4
  Constant/1 -> Multiport Switch/2
  Multiport Switch/1 -> cmd_wFault/1
  Constant1/1 -> Multiport Switch/3
  clutch_health/1 -> Multiport Switch/1

== system transmission_fault_detection/7-Speed Lepelletier/Clutch state override/Subsystem4 ==
  clutch_health : Inport
  cmd_lookup : Inport  Port=2
  Constant : Constant
  Constant1 : Constant  Value=0
  Multiport Switch : MultiPortSwitch  DataPortOrder=Specify indices  DataPortIndices={1,0,-1}  DiagnosticForDefault=None  SaturateOnIntegerOverflow=off  InputSameDT=off
  cmd_wFault : Outport
  wires:
  clutch_health/1 -> Multiport Switch/1
  Constant1/1 -> Multiport Switch/3
  Multiport Switch/1 -> cmd_wFault/1
  Constant/1 -> Multiport Switch/2
  cmd_lookup/1 -> Multiport Switch/4

== system transmission_fault_detection/7-Speed Lepelletier/Clutch state override/Subsystem5 ==
  clutch_health : Inport
  cmd_lookup : Inport  Port=2
  Constant : Constant
  Constant1 : Constant  Value=0
  Multiport Switch : MultiPortSwitch  DataPortOrder=Specify indices  DataPortIndices={1,0,-1}  DiagnosticForDefault=None  SaturateOnIntegerOverflow=off  InputSameDT=off
  cmd_wFault : Outport
  wires:
  cmd_lookup/1 -> Multiport Switch/4
  Constant/1 -> Multiport Switch/2
  Multiport Switch/1 -> cmd_wFault/1
  Constant1/1 -> Multiport Switch/3
  clutch_health/1 -> Multiport Switch/1

== system transmission_fault_detection/Fault Predictor/Detect states with matching DR/Repmat ==
  In : Inport
  Constant : Constant  Value=ones(1, numClutches )  VectorParams1D=off
  Multiply : Product  Inputs=**  Multiplication=Matrix(*)
  Out : Outport
  wires:
  Constant/1 -> Multiply/2
  In/1 -> Multiply/1
  Multiply/1 -> Out/1

== system transmission_fault_detection/Fault Predictor/|Clutch command - states table|/Repmat ==
  In1 : Inport
  Constant : Constant  Value=ones(1, length(clutch_DR_table) )  VectorParams1D=off
  Multiply1 : Product  Inputs=**  Multiplication=Matrix(*)
  Transpose : matrix_library/Transpose
  Out1 : Outport
  wires:
  Constant/1 -> Multiply1/2
  Multiply1/1 -> Transpose/1
  In1/1 -> Multiply1/1
  Transpose/1 -> Out1/1
